simulink library "tqd"  (R2021b)
settings: Solver=VariableStepAuto  StartTime=0.0  StopTime=10.0  RelTol=1e-3
undefined symbols (not defined in the file or in its folder): ATQD_APSDecReq_X_kph, ATQD_APSDecReq_Y_mps2, ATQD_APSDecReqCMD_X_kph, ATQD_APSDecReqTs_X_pct, ATQD_APSDecTimeGain_X_Deg, ATQD_APSDecTimeGain_Y_s, ATQD_APSReqLowSpd_X_Deg, ATQD_AutoHoldReleaseBPS_X_Deg, ATQD_AWDLoadTrqnsGain_X_kg, ATQD_AWDLoadTrqnsGain_Y_pct, ATQD_BOSEnBPSPosn_X_kph, ATQD_BOSMap_X_rpm, ATQD_BOSMap_Y_pct, ATQD_CreepBaseTqD_X_kph, ATQD_CreepBaseTqD_Y_Deg, ATQD_CreepBaseTqR_X_kph, ATQD_CreepBaseTqR_Y_Deg, ATQD_CreepBPSDisPosn_X_Deg, ATQD_CreepBPSDisPosnR_X_Deg, ATQD_CreepBPSEnPosn_X_Deg, ATQD_CreepBPSEnPosnR_X_Deg, ATQD_CreepDeltaTq_X_kph, ATQD_CreepIterm_X_kph, ATQD_CreepIterm_Y_kph, ATQD_CreepItermMaxLimit_X_pct, ATQD_CreepPreloadTime_X_kph, ATQD_CreepPreloadTq_X_kph, ATQD_CreepPreloadTq_Y_s, ATQD_CreepProtTq_X_Deg, ATQD_CreepPterm_X_kph, ATQD_ECOTqMapD_X_rpm, ATQD_ECOTqMapD_Y_pct, ATQD_EOPDTqMapDCon_X_rpm, ATQD_EOPDTqMapDCon_Y_Deg, ATQD_EstInitVehWeight_X_c, ATQD_LHMRollGenMapD_X_rpm, ATQD_LHMRollGenMapD_Y_rpm, ATQD_LHMTqMapD_X_rpm, ATQD_LHMTqMapD_Y_pct, ATQD_NL1TqMapD_X_rpm, ATQD_NL1TqMapD_Y_pct, ATQD_NOPDTqMapDCon_X_rpm, ATQD_NOPDTqMapDCon_Y_Deg, ATQD_NRMRrEDUSpRat_X_rpm, ATQD_NRMRrEDUSpRat_Y_Nm, ATQD_OPDHoldDownRelDelay_X_Deg, ATQD_OPDHoldEnSpd_X_Deg, ATQD_OPDHoldRelDetTime_X_Deg, ATQD_OPDHoldReleaseTq_X_Deg, ATQD_OrigPedTqLowLim_X_Deg, ATQD_OrigPedTqLowLim_Y_pct, ATQD_PedalMapClimbUpLim_X_rpm, ATQD_PedalMapClimbUpLim_Y_Deg, ATQD_PreLoadTq_X_s, ATQD_RollGenMapEL1_X_rpm, ATQD_RollGenMapEL1_Y_rpm, ATQD_SL1TqMapD_X_rpm, ATQD_SL1TqMapD_Y_pct, ATQD_SlideRegenTqGain_X_Gps, ATQD_SlideRegenTqGain_Y_pct ... (+378)
libraries: hcu_lib x59, simulink x49
(part 2 of 12)

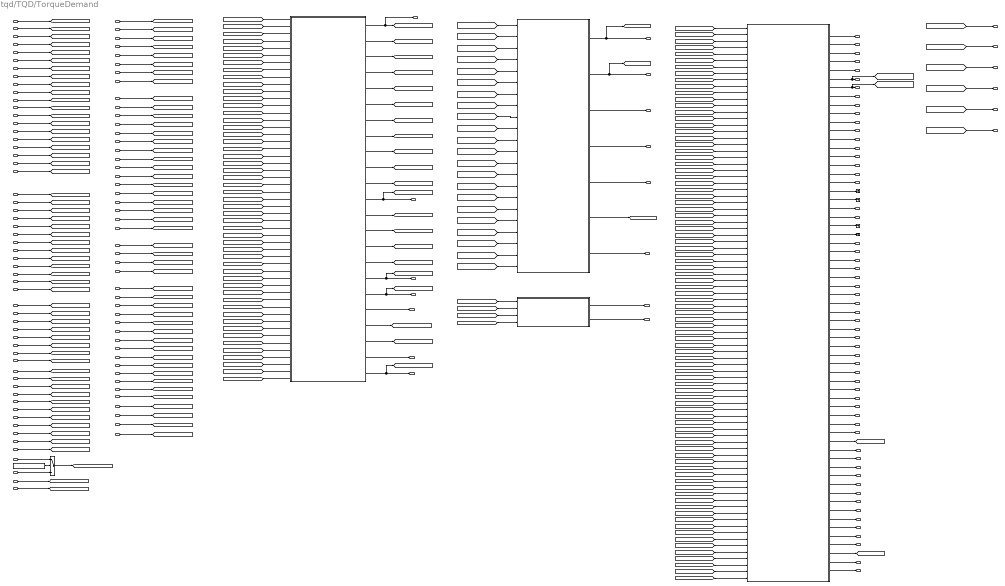
== system tqd/TQD/TorqueDemand ==
  note: Input Signals
  task_time_s : Inport
  VDHP_ActAPSPosn_pct : Inport  Port=2
  VDHP_LowIdleAccPedal_flg : Inport  Port=3
  VPMM_PowerSta_enum : Inport  Port=4
  VPMM_DrivetrainSelect_enum : Inport  Port=5
  VPMM_SysPowerMode_enum : Inport  Port=6
  VINP_VehSpeed_kph : Inport  Port=7
  VINP_BrkSwSta_flg : Inport  Port=8
  VINP_BrkSwV_flg : Inport  Port=9
  VINP_BrkPedalPos_pct : Inport  Port=10
  VINP_BrkPedalPosSta_flg : Inport  Port=11
  VINP_FrPTCSActive_flg : Inport  Port=12
  VINP_RrPTCSActive_flg : Inport  Port=13
  VINP_FrntAxlTrqReqDrv_Nm : Inport  Port=14
  VINP_RearAxlTrqReqDrv_Nm : Inport  Port=15
  VINP_FrRBCActive_flg : Inport  Port=16
  VINP_RrRBCActive_flg : Inport  Port=17
  VINP_FrntAxlTrqReqBrk_Nm : Inport  Port=18
  VINP_RearAxlTrqReqBrk_Nm : Inport  Port=19
  VINP_ADASForceIdle_flg : Inport  Port=20
  VINP_CrashOutputSts_enum : Inport  Port=21
  VINP_LongAccel_Gps : Inport  Port=22
  VINP_EPBCarWashMode_flg : Inport  Port=23
  VINP_EPBErrSta_enum : Inport  Port=24
  VINP_EPBSta_enum : Inport  Port=25
  VINP_DOASta_flg : Inport  Port=26
  VINP_HSAActive_flg : Inport  Port=27
  VINP_DriverSeatBeltCmd_flg : Inport  Port=28
  VINP_AVHActive_flg : Inport  Port=29
  VINP_ACCRequiredAccel_mps2 : Inport  Port=30
  VINP_ACCVehHoldReq_flg : Inport  Port=31
  VINP_PsngrSeatBeltCmd_flg : Inport  Port=32
  VINP_RDriverSeatBeltCmd_flg : Inport  Port=33
  VINP_RCenterSeatBeltCmd_flg : Inport  Port=34
  VINP_RPsngrSeatBeltCmd_flg : Inport  Port=35
  VINP_SASAngle_Deg : Inport  Port=36
  VINP_YawRate_degps : Inport  Port=37
  VINP_ADASACCSta_enum : Inport  Port=38
  VINP_ABSActive_flg : Inport  Port=39
  VINP_ESCActive_flg : Inport  Port=40
  VINP_IVIPWModeReq_enum : Inport  Port=41
  VINP_IVICreepSWReq_flg : Inport  Port=42
  VINP_RollModeSWCmd_enum : Inport  Port=43
  VINP_IVIPwrLockSW_enum : Inport  Port=44
  VINP_ShifterHandleCmd_enum : Inport  Port=45
  VINP_FrEDURotateDirction_enum : Inport  Port=46
  VINP_RrEDURotateDirction_enum : Inport  Port=47
  VINP_FrTMSpd_RPM : Inport  Port=48
  VINP_RrTMSpd_RPM : Inport  Port=49
  VINP_HVBPwrAvailDchrg_kw : Inport  Port=50
  VINP_HVBPwrAvailChrg_kw : Inport  Port=51
  VINP_FrRegenAvailTq_Nm : Inport  Port=52
  VINP_RrRegenAvailTq_Nm : Inport  Port=53
  VINP_FrEDURealTMTq_Nm : Inport  Port=54
  VINP_RrEDURealTMTq_Nm : Inport  Port=55
  VINP_HVBattErr_flg : Inport  Port=56
  VINP_DCDCFaultSta_enum : Inport  Port=57
  VINP_FrMotorAvailTq_Nm : Inport  Port=58
  VINP_RrMotorAvailTq_Nm : Inport  Port=59
  VINP_MCUWarnF_enum : Inport  Port=60
  VINP_MCUWarnR_enum : Inport  Port=61
  VINP_ChrgPlugSta_enum : Inport  Port=62
  VINP_HVBattSOC_pct : Inport  Port=63
  VINP_RegenMode_enum : Inport  Port=64
  VINP_DrSCPSysErrLmp_enum : Inport  Port=65
  VINP_SCPSystemMode_enum : Inport  Port=66
  VVMC_ADASActive_flg : Inport  Port=67
  VVMC_ADASWhlTqReq_Nm : Inport  Port=68
  VVMC_CruzActive_flg : Inport  Port=69
  VVMC_CruzWhlTqReq_Nm : Inport  Port=70
  VVMC_MSAActive_flg : Inport  Port=71
  VVMC_MSAWhlTqReq_Nm : Inport  Port=72
  VVMC_APSActive_flg : Inport  Port=73
  VVMC_APSSpeedCMD_kph : Inport  Port=74
  VVMC_APSShiftPosnReq_enum : Inport  Port=75
  VVMC_ACCPedalOvrd_flg : Inport  Port=76
  VVMC_LongAcc_Gps : Inport  Port=77
  VVMC_ActMaxSlideRate_pct : Inport  Port=78
  VVMC_EstSlope_Deg : Inport  Port=79
  VVMC_APSReq_enum : Inport  Port=80
  VVMC_RWDRDCActive_enum : Inport  Port=81
  VVMC_ActLRSlideRate_pct : Inport  Port=82
  VVMC_ActRRSlideRate_pct : Inport  Port=83
  VVMC_ActStESCYaw_degps : Inport  Port=84
  VVMC_CAASActive_flg : Inport  Port=85
  VVMC_CalibratedGyroY_Dps : Inport  Port=86
  VINP_BrakeSWGPIO_flg : Inport  Port=87
  VINP_CrashSignalGPIO_flg : Inport  Port=88
  VINP_DrDoorSW_flg : Inport  Port=89
  VINP_SeatSW_flg : Inport  Port=90
  VINP_HoodSW_flg : Inport  Port=91
  VINP_TailgateSW_flg : Inport  Port=92
  VINP_PsDoorSW_flg : Inport  Port=93
  VINP_RRDoorSW_flg : Inport  Port=94
  VINP_RLDoorSW_flg : Inport  Port=95
  VTQR_ActualFEDUWhlTqReq_Nm : Inport  Port=96
  VTQR_ActualREDUWhlTqReq_Nm : Inport  Port=97
  VTQR_NoABSFEDUWhlTqReq_Nm : Inport  Port=98
  VTQR_NoABSREDUWhlTqReq_Nm : Inport  Port=99
  VINP_PBWMotorPos_enum : Inport  Port=100
  VDDM_LimpHomeAct_flg : Inport  Port=101
  VINP_CreepSW_flg : Inport  Port=102
  Constant21 : Constant  Value=KTQD_YawRateSW_flg
  CrashDetect : Subsystem
  ShiftModule : Subsystem
      settings: AttributesFormatString=Priority%<Priority>
  Signal_convert : Subsystem
  Switch : Switch  Criteria=u2 > Threshold
  Terminator{,1..3} (4 alike) : Terminator
  TorqueModule : Subsystem
      settings: AttributesFormatString=Priority%<Priority>
  VTQD_GearActualPosn_enum : Outport
  VTQD_ParkRequest_flg : Outport  Port=2
  VTQD_PBWLockTO_flg : Outport  Port=3
  VTQD_PBWUnlockTO_flg : Outport  Port=4
  VTQD_DriverWhlTqDem_Nm : Outport  Port=5
  VTQD_AfterAvailableTqDemFr_Nm : Outport  Port=6
  VTQD_AfterAvailableTqDemRr_Nm : Outport  Port=7
  VTQD_TqSourceFr_enum : Outport  Port=8
  VTQD_TqSourceRr_enum : Outport  Port=9
  VTQD_FrEDUAvailBrkRgnTq_Nm : Outport  Port=10
  VTQD_RrEDUAvailBrkRgnTq_Nm : Outport  Port=11
  VTQD_TqTargetShaftSpd_rpm : Outport  Port=12
  VTQD_LimpHomeAct_flg : Outport  Port=13
  VTQD_RollRegenEnable_flg : Outport  Port=14
  VTQD_EVDriveMode_enum : Outport  Port=15
  VTQD_EVDriveModeValid_flg : Outport  Port=16
  VTQD_ShiftGearPosn_enum : Outport  Port=17
  VTQD_PButtonSta_enum : Outport  Port=18
  VTQD_FrActvDmpDisabReq_flg : Outport  Port=19
  VTQD_RrActvDmpDisabReq_flg : Outport  Port=20
  VTQD_FrRgnDecrSta_flg : Outport  Port=21
  VTQD_RrRgnDecrSta_flg : Outport  Port=22
  VTQD_DriverWhlTqDemFr_Nm : Outport  Port=23
  VTQD_DriverWhlTqDemRr_Nm : Outport  Port=24
  VTQD_FrEDUActTq_Nm : Outport  Port=25
  VTQD_RrEDUActTq_Nm : Outport  Port=26
  VTQD_FrEDURolRgnTq_Nm : Outport  Port=27
  VTQD_RrEDURolRgnTq_Nm : Outport  Port=28
  VTQD_FrEDUSpd_rpm : Outport  Port=29
  VTQD_RrEDUSpd_rpm : Outport  Port=30
  VTQD_FrEDUSpdValid_flg : Outport  Port=31
  VTQD_FrEDUAvailBrkRgnTqV_flg : Outport  Port=32
  VTQD_RrEDUSpdValid_flg : Outport  Port=33
  VTQD_RrEDUAvailBrkRgnTqV_flg : Outport  Port=34
  VTQD_RgnAbnorSta_flg : Outport  Port=35
  VTQD_PTCSPermSta_flg : Outport  Port=36
  VTQD_FrRgnPermSta_flg : Outport  Port=37
  VTQD_RrRgnPermSta_flg : Outport  Port=38
  VTQD_ExternalTqAllow_flg : Outport  Port=39
  VTQD_FrIdcMin_A : Outport  Port=40
  VTQD_FrIdcMax_A : Outport  Port=41
  VTQD_FrUdcMin_V : Outport  Port=42
  VTQD_FrUdcMax_V : Outport  Port=43
  VTQD_RrIdcMin_A : Outport  Port=44
  VTQD_RrIdcMax_A : Outport  Port=45
  VTQD_RrUdcMin_V : Outport  Port=46
  VTQD_RrUdcMax_V : Outport  Port=47
  VTQD_CoordWhlTqDemFr_Nm : Outport  Port=48
  VTQD_CoordWhlTqDemRr_Nm : Outport  Port=49
  VTQD_CreepEnable_flg : Outport  Port=50
  VTQD_CrashDetd_flg : Outport  Port=51
  VTQD_DiagHCrash_flg : Outport  Port=52
  VTQD_ReBrakeLPReq_flg : Outport  Port=53
  VTQD_LoSpdBrkCtrl_flg : Outport  Port=54
  VTQD_LowIdleAccPedal_flg : Outport  Port=55
  VTQD_APSStaSys_enum : Outport  Port=56
  VTQD_APSReq_enum : Outport  Port=57
  VTQD_APSDecReqA_flg : Outport  Port=58
  VTQD_APSDecReq_mps2 : Outport  Port=59
  VTQD_ExtShftAllow_flg : Outport  Port=60
  VTQD_EstVehWeightResult_kg : Outport  Port=61
  VTQD_BOSEnable_flg : Outport  Port=62
  VTQD_CreepON_flg : Outport  Port=63
  VTQD_PreLoadHold_flg : Outport  Port=64
  VTQD_PreLoadPreEn_flg : Outport  Port=65
  VTQD_CreepPrLoadEnable_flg : Outport  Port=66
  VTQD_RDCActive_enum : Outport  Port=67
  VTQD_EquivAccPedalSWSta_flg : Outport  Port=68
  VTQD_DriveProtEn_flg : Outport  Port=69
  VTQD_ActParkRequest_flg : Outport  Port=70
  VTQD_RegenTqLimitEn_flg : Outport  Port=71
  VTQD_PedAccTqEn_flg : Outport  Port=72
  VTQD_IVIPwrLockSta_enum : Outport  Port=73
  VTQD_ExtDoorAllow_flg : Outport  Port=74
  VTQD_OPDHoldLamp_flg : Outport  Port=75
  VTQD_RegenMode_enum : Outport  Port=76
  VTQD_VehActSpd_kph : Outport  Port=77
  VTQD_CreepBaseTqD_Nm : Outport  Port=78
  wires:
  VINP_FrTMSpd_RPM/1 -> [VINP_FrTMSpd_rpm]
  VDHP_ActAPSPosn_pct/1 -> [VDHP_ActAPSPosn_pct]
  VPMM_PowerSta_enum/1 -> [VPMM_PowerSta_enum]
  task_time_s/1 -> [task_time_s]
  VINP_VehSpeed_kph/1 -> [VINP_VehSpeed_kph]
  VINP_BrkSwSta_flg/1 -> [VINP_BrkSwSta_flg]
  VINP_ShifterHandleCmd_enum/1 -> [VINP_ShifterHandleCmd_enum]
  VDHP_LowIdleAccPedal_flg/1 -> [VDHP_LowIdleAccPedal_flg]
  VINP_PBWMotorPos_enum/1 -> [VINP_PBWMotorPos_enum]
  Signal_convert/8(VTQD_TqTargetShaftSpd_rpm) -> [VTQD_TqTargetShaftSpd_rpm]
  Signal_convert/2(VTQD_RollRegenDisable_flg) -> [VTQD_RollRegenDisableReq_flg]
  Signal_convert/5(VTQD_ActBPSPosn_pct) -> [VTQD_ActBPSPosn_pct]
  Signal_convert/11(VTQD_EVDriveMode_enum) -> [VTQD_EVDriveMode_enum]
  Signal_convert/10(VTQD_LimpHomeAct_flg) -> [VTQD_LimpHomeAct_flg]
  Signal_convert/12(VTQD_CreepON_flg) -> [VTQD_CreepON_flg], VTQD_CreepON_flg/1
  [VTQD_TMRotateDirction_enum] -> ShiftModule/7(VTQD_TMRotateDirction_enum)
  ShiftModule/4(VTQD_PBWUnlockTO_flg) -> VTQD_PBWUnlockTO_flg/1
  [VINP_VehSpeed_kph] -> ShiftModule/3(VINP_VehSpeed_kph)
  [VPMM_PowerSta_enum] -> ShiftModule/5(VPMM_PowerSta_enum)
  [task_time_s] -> ShiftModule/1(task_time_s)
  [VTQD_BrkSwSta_flg] -> ShiftModule/4(VTQD_BrkSwSta_flg)
  ShiftModule/2(VTQD_ParkRequest_flg) -> [VTQD_ParkRequest_flg], VTQD_ParkRequest_flg/1
  [VINP_ShifterHandleCmd_enum] -> ShiftModule/2(VINP_ShifterHandleCmd_enum)
  ShiftModule/3(VTQD_PBWLockTO_flg) -> VTQD_PBWLockTO_flg/1
  [VINP_PBWMotorPos_enum] -> ShiftModule/6(VINP_PBWMotorPos_enum)
  ShiftModule/1(VTQD_GearActualPosn_enum) -> [VTQD_GearActualPosn_enum], VTQD_GearActualPosn_enum/1
  [VTQD_RollRegenDisableReq_flg] -> TorqueModule/3(VTQD_RollRegenDisableReq_flg)
  [VTQD_GearActualPosn_enum] -> TorqueModule/4(VTQD_GearActualPosn_enum)
  [VTQD_CreepON_flg] -> TorqueModule/5(VTQD_CreepON_flg)
  [VTQD_BrkSwSta_flg] -> TorqueModule/6(VTQD_BrkSwSta_flg)
  [VINP_FrntAxlTrqReqBrk_Nm] -> TorqueModule/22(VINP_FrntAxlTrqReqBrk_Nm)
  [VINP_RearAxlTrqReqBrk_Nm] -> TorqueModule/23(VINP_RearAxlTrqReqBrk_Nm)
  [VINP_RearAxlTrqReqDrv_Nm] -> TorqueModule/19(VINP_RearAxlTrqReqDrv_Nm)
  [VINP_FrntAxlTrqReqDrv_Nm] -> TorqueModule/18(VINP_FrntAxlTrqReqDrv_Nm)
  [VTQD_LimpHomeAct_flg] -> TorqueModule/7(VTQD_LimpHomeAct_flg)
  [VINP_VehSpeed_kph] -> TorqueModule/10(VINP_VehSpeed_kph)
  [VTQD_TqTargetShaftSpd_rpm] -> TorqueModule/11(VTQD_TqTargetShaftSpd_rpm)
  [VTQD_ActBPSPosn_pct] -> TorqueModule/15(VTQD_ActBPSPosn_pct)
  [VVMC_APSActive_flg] -> TorqueModule/30(VVMC_APSActive_flg)
  [VVMC_ADASActive_flg] -> TorqueModule/24(VVMC_ADASActive_flg)
  [VVMC_ADASWhlTqReq_Nm] -> TorqueModule/25(VVMC_ADASWhlTqReq_Nm)
  [VVMC_CruzActive_flg] -> TorqueModule/26(VVMC_CruzActive_flg)
  [VVMC_CruzWhlTqReq_Nm] -> TorqueModule/27(VVMC_CruzWhlTqReq_Nm)
  [VVMC_MSAActive_flg] -> TorqueModule/28(VVMC_MSAActive_flg)
  [VVMC_MSAWhlTqReq_Nm] -> TorqueModule/29(VVMC_MSAWhlTqReq_Nm)
  VINP_HVBPwrAvailDchrg_kw/1 -> [VINP_HVBPwrAvailDchrg_kw]
  VINP_HVBPwrAvailChrg_kw/1 -> [VINP_HVBPwrAvailChrg_kw]
  [VINP_HVBPwrAvailDchrg_kw] -> TorqueModule/31(VINP_HVBPwrAvailDchrg_kw)
  [VINP_HVBPwrAvailChrg_kw] -> TorqueModule/34(VINP_HVBPwrAvailChrg_kw)
  [VINP_CreepSW_flg] -> Signal_convert/15(VINP_CreepSW_flg)
  VINP_CreepSW_flg/1 -> [VINP_CreepSW_flg]
  VDDM_LimpHomeAct_flg/1 -> [VDDM_LimpHomeAct_flg]
  [VDDM_LimpHomeAct_flg] -> Signal_convert/14(VDDM_LimpHomeAct_flg)
  VINP_BrkSwV_flg/1 -> [VINP_BrkSwV_flg]
  VINP_FrPTCSActive_flg/1 -> [VINP_FrPTCSActive_flg]
  VINP_FrntAxlTrqReqDrv_Nm/1 -> [VINP_FrntAxlTrqReqDrv_Nm]
  VINP_RearAxlTrqReqDrv_Nm/1 -> [VINP_RearAxlTrqReqDrv_Nm]
  VINP_FrRBCActive_flg/1 -> [VINP_FrRBCActive_flg]
  VINP_FrntAxlTrqReqBrk_Nm/1 -> [VINP_FrntAxlTrqReqBrk_Nm]
  VINP_RearAxlTrqReqBrk_Nm/1 -> [VINP_RearAxlTrqReqBrk_Nm]
  VINP_BrkPedalPos_pct/1 -> [VINP_BrkPedalPos_pct]
  VINP_BrkPedalPosSta_flg/1 -> [VINP_BrkPedalPosSta_flg]
  [VINP_BrkSwSta_flg] -> Signal_convert/4(VINP_BrkSwSta_flg)
  [VINP_BrkSwV_flg] -> Signal_convert/6(VINP_BrkSwV_flg)
  [VINP_BrkPedalPos_pct] -> Signal_convert/7(VINP_BrkPedalPos_pct)
  [VINP_BrkPedalPosSta_flg] -> Signal_convert/8(VINP_BrkPedalPosSta_flg)
  [VTQD_TqTargetShaftSpd_rpm] -> VTQD_TqTargetShaftSpd_rpm/1
  [VTQD_LowIdleAccPedal_flg] -> TorqueModule/1(VTQD_LowIdleAccPedal_flg)
  [VPMM_DrivetrainSelect_enum] -> TorqueModule/2(VPMM_DrivetrainSelect_enum)
  VINP_RrTMSpd_RPM/1 -> [VINP_RrTMSpd_rpm]
  [VPMM_DrivetrainSelect_enum] -> Signal_convert/11(VPMM_DrivetrainSelect_enum)
  VPMM_DrivetrainSelect_enum/1 -> [VPMM_DrivetrainSelect_enum]
  [VDHP_ActAPSPosn_pct] -> Signal_convert/3(VDHP_ActAPSPosn_pct)
  Signal_convert/3(VTQD_ActAPSPosn_pct) -> [VTQD_ActAPSPosn_pct]
  [VTQD_ActAPSPosn_pct] -> TorqueModule/14(VTQD_ActAPSPosn_pct)
  [VTQD_GearActualPosn_enum] -> Signal_convert/1(VTQD_GearActualPosn_enum)
  [VINP_FrTMSpd_rpm] -> Signal_convert/9(VINP_FrTMSpd_rpm)
  [VINP_RrTMSpd_rpm] -> Signal_convert/10(VINP_RrTMSpd_rpm)
  VINP_FrEDURotateDirction_enum/1 -> [VINP_FrEDURotateDirction_enum]
  VINP_RrEDURotateDirction_enum/1 -> [VINP_RrEDURotateDirction_enum]
  [VINP_RrEDURotateDirction_enum] -> Signal_convert/13(VINP_RrEDURotateDirction_enum)
  [VINP_FrEDURotateDirction_enum] -> Signal_convert/12(VINP_FrEDURotateDirction_enum)
  Signal_convert/6(VTQD_FrShaftSpd_rpm) -> [VTQD_FrShaftSpd_rpm]
  Signal_convert/7(VTQD_RrShaftSpd_rpm) -> [VTQD_RrShaftSpd_rpm]
  Signal_convert/9(VTQD_TMRotateDirction_enum) -> [VTQD_TMRotateDirction_enum]
  Signal_convert/4(VTQD_BrkSwSta_flg) -> [VTQD_BrkSwSta_flg]
  [VTQD_FrShaftSpd_rpm] -> TorqueModule/12(VTQD_FrShaftSpd_rpm)
  [VTQD_RrShaftSpd_rpm] -> TorqueModule/13(VTQD_RrShaftSpd_rpm)
  Signal_convert/1(VTQD_LowIdleAccPedal_flg) -> VTQD_LowIdleAccPedal_flg/1, [VTQD_LowIdleAccPedal_flg]
  [VDHP_LowIdleAccPedal_flg] -> Signal_convert/2(VDHP_LowIdleAccPedal_flg)
  [VTQD_LimpHomeAct_flg] -> VTQD_LimpHomeAct_flg/1
  [VTQD_EVDriveMode_enum] -> VTQD_EVDriveMode_enum/1
  VINP_BrakeSWGPIO_flg/1 -> [VINP_BrakeSWGPIO_flg]
  [VINP_BrakeSWGPIO_flg] -> Signal_convert/5(VINP_BrakeSWGPIO_flg)
  Signal_convert/13(VTQD_ShiftGearPosn_enum) -> [VTQD_ShiftGearPosn_enum]
  [VTQD_ShiftGearPosn_enum] -> VTQD_ShiftGearPosn_enum/1
  ShiftModule/5(VTQD_PButtonSta_enum) -> VTQD_PButtonSta_enum/1
  [VINP_VehSpeed_kph] -> Signal_convert/16(VINP_VehSpeed_kph)
  Signal_convert/14(VTQD_FrActvDmpDisabReq_flg) -> [VTQD_FrActvDmpDisabReq_flg]
  Signal_convert/15(VTQD_RrActvDmpDisabReq_flg) -> [VTQD_RrActvDmpDisabReq_flg]
  [VTQD_FrActvDmpDisabReq_flg] -> VTQD_FrActvDmpDisabReq_flg/1
  [VTQD_RrActvDmpDisabReq_flg] -> VTQD_RrActvDmpDisabReq_flg/1
  VINP_RrPTCSActive_flg/1 -> [VINP_RrPTCSActive_flg]
  [VINP_FrPTCSActive_flg] -> TorqueModule/16(VINP_FrPTCSActive_flg)
  [VINP_RrPTCSActive_flg] -> TorqueModule/17(VINP_RrPTCSActive_flg)
  VINP_RrRBCActive_flg/1 -> [VINP_RrRBCActive_flg]
  [VINP_FrRBCActive_flg] -> TorqueModule/20(VINP_FrRBCActive_flg)
  [VINP_RrRBCActive_flg] -> TorqueModule/21(VINP_RrRBCActive_flg)
  VINP_RrRegenAvailTq_Nm/1 -> [VINP_RrRegenAvailTq_Nm]
  VINP_FrEDURealTMTq_Nm/1 -> [VINP_FrEDURealTMTq_Nm]
  VINP_FrRegenAvailTq_Nm/1 -> [VINP_FrRegenAvailTq_Nm]
  VINP_RrEDURealTMTq_Nm/1 -> [VINP_RrEDURealTMTq_Nm]
  [VINP_FrRegenAvailTq_Nm] -> TorqueModule/35(VINP_FrRegenAvailTq_Nm)
  [VINP_RrRegenAvailTq_Nm] -> TorqueModule/36(VINP_RrRegenAvailTq_Nm)
  [VINP_FrTMSpd_rpm] -> TorqueModule/37(VINP_FrTMSpd_RPM)
  [VINP_RrTMSpd_rpm] -> TorqueModule/38(VINP_RrTMSpd_RPM)
  [VINP_FrEDURealTMTq_Nm] -> TorqueModule/39(VINP_FrEDURealTMTq_Nm)
  [VINP_RrEDURealTMTq_Nm] -> TorqueModule/40(VINP_RrEDURealTMTq_Nm)
  [VTQD_ParkRequest_flg] -> TorqueModule/41(VTQD_ParkRequest_flg)
  Signal_convert/16(VTQD_MCUReady4Ext_flg) -> [VTQD_MCUReady4Ext_flg]
  [VPMM_PowerSta_enum] -> TorqueModule/42(VPMM_PwrSta_enum)
  [VTQD_MCUReady4Ext_flg] -> TorqueModule/43(VTQD_MCUReady4Ext_flg)
  VINP_DCDCFaultSta_enum/1 -> [VINP_DCDCFaultSta_enum]
  VINP_ADASForceIdle_flg/1 -> [VINP_ADASForceIdle_flg]
  VINP_HVBattErr_flg/1 -> [VINP_HVBattErr_flg]
  [VINP_HVBattErr_flg] -> TorqueModule/44(VINP_HVBattErr_flg)
  [VINP_DCDCFaultSta_enum] -> TorqueModule/45(VINP_DCDCFaultSta_enum)
  [VINP_ADASForceIdle_flg] -> TorqueModule/46(VINP_ADASForceIdle_flg)
  VVMC_ADASActive_flg/1 -> [VVMC_ADASActive_flg]
  VVMC_ADASWhlTqReq_Nm/1 -> [VVMC_ADASWhlTqReq_Nm]
  VVMC_APSActive_flg/1 -> [VVMC_APSActive_flg]
  [VTQD_TMRotateDirction_enum] -> TorqueModule/47(VTQD_TMRotateDirction_enum)
  VINP_IVIPWModeReq_enum/1 -> [VINP_IVIPWModeReq_enum]
  VINP_RegenMode_enum/1 -> [VINP_RegenMode_enum]
  [VTQD_EVDriveMode_enum] -> TorqueModule/8(VTQD_EVDriveMode_enum)
  [VTQD_RegenMode_enum] -> TorqueModule/9(VTQD_RegenMode_enum)
  TorqueModule/1(VTQD_DriverWhlTqDem_Nm) -> VTQD_DriverWhlTqDem_Nm/1
  TorqueModule/2(VTQD_TqSourceFr_enum) -> VTQD_TqSourceFr_enum/1
  TorqueModule/3(VTQD_TqSourceRr_enum) -> VTQD_TqSourceRr_enum/1  "VTQD_TqSourceRr_enum"
  TorqueModule/4(VTQD_RollRegenEnable_flg) -> VTQD_RollRegenEnable_flg/1
  TorqueModule/5(VTQD_EVDriveModeValid_flg) -> VTQD_EVDriveModeValid_flg/1
  TorqueModule/6(VTQD_AfterAvailableTqDemFr_Nm) -> [VTQD_AfterAvailableTqDemFr_Nm], VTQD_AfterAvailableTqDemFr_Nm/1
  TorqueModule/7(VTQD_AfterAvailableTqDemRr_Nm) -> [VTQD_AfterAvailableTqDemRr_Nm], VTQD_AfterAvailableTqDemRr_Nm/1
  TorqueModule/8(VTQD_FrEDUAvailBrkRgnTq_Nm) -> VTQD_FrEDUAvailBrkRgnTq_Nm/1
  TorqueModule/9(VTQD_RrEDUAvailBrkRgnTq_Nm) -> VTQD_RrEDUAvailBrkRgnTq_Nm/1
  TorqueModule/10(VTQD_FrRgnDecrSta_flg) -> VTQD_FrRgnDecrSta_flg/1
  TorqueModule/11(VTQD_RrRgnDecrSta_flg) -> VTQD_RrRgnDecrSta_flg/1
  TorqueModule/12(VTQD_FrEDUActTq_Nm) -> VTQD_FrEDUActTq_Nm/1
  TorqueModule/13(VTQD_RrEDUActTq_Nm) -> VTQD_RrEDUActTq_Nm/1
  TorqueModule/14(VTQD_FrEDURolRgnTq_Nm) -> VTQD_FrEDURolRgnTq_Nm/1
  TorqueModule/15(VTQD_RrEDURolRgnTq_Nm) -> VTQD_RrEDURolRgnTq_Nm/1
  TorqueModule/16(VTQD_FrEDUSpd_rpm) -> VTQD_FrEDUSpd_rpm/1
  TorqueModule/17(VTQD_RrEDUSpd_rpm) -> VTQD_RrEDUSpd_rpm/1
  TorqueModule/18(VTQD_FrEDUSpdValid_flg) -> VTQD_FrEDUSpdValid_flg/1
  TorqueModule/21(VTQD_FrEDUAvailBrkRgnTqV_flg) -> VTQD_FrEDUAvailBrkRgnTqV_flg/1
  TorqueModule/22(VTQD_RrEDUSpdValid_flg) -> VTQD_RrEDUSpdValid_flg/1
  TorqueModule/23(VTQD_RrEDUActTqValid_flg) -> Terminator2/1
  TorqueModule/24(VTQD_RrEDURolRgnTqValid_flg) -> Terminator3/1
  TorqueModule/25(VTQD_RrEDUAvailBrkRgnTqV_flg) -> VTQD_RrEDUAvailBrkRgnTqV_flg/1
  TorqueModule/26(VTQD_RgnAbnorSta_flg) -> VTQD_RgnAbnorSta_flg/1
  TorqueModule/27(VTQD_PTCSPermSta_flg) -> VTQD_PTCSPermSta_flg/1
  TorqueModule/28(VTQD_FrRgnPermSta_flg) -> VTQD_FrRgnPermSta_flg/1
  TorqueModule/29(VTQD_RrRgnPermSta_flg) -> VTQD_RrRgnPermSta_flg/1
  TorqueModule/30(VTQD_DriverWhlTqDemFr_Nm) -> VTQD_DriverWhlTqDemFr_Nm/1
  TorqueModule/31(VTQD_DriverWhlTqDemRr_Nm) -> VTQD_DriverWhlTqDemRr_Nm/1
  TorqueModule/32(VTQD_ExternalTqAllow_flg) -> VTQD_ExternalTqAllow_flg/1
  TorqueModule/33(VTQD_FrIdcMin_A) -> VTQD_FrIdcMin_A/1
  TorqueModule/34(VTQD_FrIdcMax_A) -> VTQD_FrIdcMax_A/1
  TorqueModule/35(VTQD_FrUdcMin_V) -> VTQD_FrUdcMin_V/1
  TorqueModule/36(VTQD_FrUdcMax_V) -> VTQD_FrUdcMax_V/1
  TorqueModule/37(VTQD_RrIdcMin_A) -> VTQD_RrIdcMin_A/1
  TorqueModule/38(VTQD_RrIdcMax_A) -> VTQD_RrIdcMax_A/1
  TorqueModule/39(VTQD_RrUdcMin_V) -> VTQD_RrUdcMin_V/1
  TorqueModule/40(VTQD_RrUdcMax_V) -> VTQD_RrUdcMax_V/1
  TorqueModule/41(VTQD_CoordWhlTqDemFr_Nm) -> VTQD_CoordWhlTqDemFr_Nm/1
  TorqueModule/42(VTQD_CoordWhlTqDemRr_Nm) -> VTQD_CoordWhlTqDemRr_Nm/1
  TorqueModule/43(VTQD_CreepEnable_flg) -> VTQD_CreepEnable_flg/1
  [VINP_IVIPWModeReq_enum] -> Signal_convert/17(VINP_IVIPWModeReq_enum)
  VVMC_CruzActive_flg/1 -> [VVMC_CruzActive_flg]
  VVMC_CruzWhlTqReq_Nm/1 -> [VVMC_CruzWhlTqReq_Nm]
  VVMC_MSAActive_flg/1 -> [VVMC_MSAActive_flg]
  VVMC_MSAWhlTqReq_Nm/1 -> [VVMC_MSAWhlTqReq_Nm]
  VINP_CrashSignalGPIO_flg/1 -> [VINP_CrashSignalGPIO_flg]
  VINP_CrashOutputSts_enum/1 -> [VINP_CrashOutputSts_enum]
  CrashDetect/1(VTQD_CrashDetd_flg) -> VTQD_CrashDetd_flg/1  "VTQD_CrashDetd_flg"
  CrashDetect/2(VTQD_DiagHCrash_flg) -> VTQD_DiagHCrash_flg/1  "VTQD_DiagHCrash_flg"
  VINP_LongAccel_Gps/1 -> [VINP_LongAccel_Gps]
  [VINP_LongAccel_Gps] -> TorqueModule/48(VINP_LongAccel_Gps)
  TorqueModule/44(VTQD_ReBrakeLPReq_flg) -> VTQD_ReBrakeLPReq_flg/1
  VTQR_ActualFEDUWhlTqReq_Nm/1 -> [VTQR_ActualFEDUWhlTqReq_Nm]
  VTQR_ActualREDUWhlTqReq_Nm/1 -> [VTQR_ActualREDUWhlTqReq_Nm]
  [VTQR_ActualFEDUWhlTqReq_Nm] -> TorqueModule/49(VTQR_ActualFEDUWhlTqReq_Nm)
  [VTQR_ActualREDUWhlTqReq_Nm] -> TorqueModule/50(VTQR_ActualREDUWhlTqReq_Nm)
  [VTQD_RDCActive_enum] -> TorqueModule/51(VTQD_RDCActive_enum)
  VINP_EPBCarWashMode_flg/1 -> [VINP_EPBCarWashMode_flg]
  VINP_EPBErrSta_enum/1 -> [VINP_EPBErrSta_enum]
  VINP_EPBSta_enum/1 -> [VINP_EPBSta_enum]
  VINP_DOASta_flg/1 -> [VINP_DOASta_flg]
  VINP_FrMotorAvailTq_Nm/1 -> [VINP_FrMotorAvailTq_Nm]
  VINP_RrMotorAvailTq_Nm/1 -> [VINP_RrMotorAvailTq_Nm]
  [VINP_FrMotorAvailTq_Nm] -> TorqueModule/53(VINP_FrMotorAvailTq_Nm)
  [VINP_RrMotorAvailTq_Nm] -> TorqueModule/54(VINP_RrMotorAvailTq_Nm)
  [task_time_s] -> TorqueModule/55(task_time_s)
  TorqueModule/45(VTQD_LoSpdBrkCtrl_flg) -> VTQD_LoSpdBrkCtrl_flg/1
  TorqueModule/46(VTQD_BOSEnable_flg) -> VTQD_BOSEnable_flg/1
  TorqueModule/52(VTQD_APSStaSys_enum) -> VTQD_APSStaSys_enum/1
  TorqueModule/53(VTQD_APSReq_enum) -> VTQD_APSReq_enum/1
  TorqueModule/54(VTQD_APSDecReqA_flg) -> VTQD_APSDecReqA_flg/1
  TorqueModule/55(VTQD_APSDecReq_mps2) -> VTQD_APSDecReq_mps2/1
  VINP_HSAActive_flg/1 -> [VINP_HSAActive_flg]
  VTQR_NoABSREDUWhlTqReq_Nm/1 -> [VTQR_NoABSREDUWhlTqReq_Nm]
  VTQR_NoABSFEDUWhlTqReq_Nm/1 -> [VTQR_NoABSFEDUWhlTqReq_Nm]
  VINP_AVHActive_flg/1 -> [VINP_AVHActive_flg]
  VINP_DrDoorSW_flg/1 -> [VINP_DrDoorSW_flg]
  VINP_MCUWarnF_enum/1 -> [VINP_MCUWarnF_enum]
  VINP_MCUWarnR_enum/1 -> [VINP_MCUWarnR_enum]
  VVMC_APSSpeedCMD_kph/1 -> [VVMC_APSSpeedCMD_kph]
  VVMC_APSShiftPosnReq_enum/1 -> [VVMC_APSShiftPosnReq_enum]
  VINP_DriverSeatBeltCmd_flg/1 -> [VINP_DriverSeatBeltCmd_flg]
  VINP_ChrgPlugSta_enum/1 -> [VINP_ChrgPlugSta_enum]
  VINP_SeatSW_flg/1 -> [VINP_SeatSW_flg]
  [VINP_MCUWarnF_enum] -> Signal_convert/18(VINP_MCUWarnF_enum)
  [task_time_s] -> Signal_convert/20(task_time_s)
  [VINP_FrEDURealTMTq_Nm] -> Signal_convert/21(VINP_FrEDURealTMTq_Nm)
  [VINP_RrEDURealTMTq_Nm] -> Signal_convert/22(VINP_RrEDURealTMTq_Nm)
  [VINP_MCUWarnR_enum] -> Signal_convert/19(VINP_MCUWarnR_enum)
  [VINP_HSAActive_flg] -> TorqueModule/56(VINP_HSAActive_flg)
  [VTQR_NoABSFEDUWhlTqReq_Nm] -> TorqueModule/57(VTQR_NoABSFEDUWhlTqReq_Nm)
  [VTQR_NoABSREDUWhlTqReq_Nm] -> TorqueModule/58(VTQR_NoABSREDUWhlTqReq_Nm)
  [VINP_AVHActive_flg] -> TorqueModule/59(VINP_AVHActive_flg)
  [VINP_EPBErrSta_enum] -> TorqueModule/60(VINP_EPBErrSta_enum)
  [VINP_MCUWarnF_enum] -> TorqueModule/62(VINP_MCUWarnF_enum)
  [VINP_MCUWarnR_enum] -> TorqueModule/63(VINP_MCUWarnR_enum)
  Signal_convert/17(VTQD_EstVehWeightResult_kg) -> [VTQD_EstVehWeightResult_kg], VTQD_EstVehWeightResult_kg/1
  [VTQD_EPBCarWashMode_flg] -> ShiftModule/8(VTQD_EPBCarWashMode_flg)
  [VINP_DrDoorSW_flg] -> ShiftModule/9(VINP_DrDoorSW_flg)
  [VVMC_APSShiftPosnReq_enum] -> ShiftModule/10(VVMC_APSShiftPosnReq_enum)
  [VVMC_APSActive_flg] -> ShiftModule/11(VVMC_APSActive_flg)
  [VINP_DriverSeatBeltCmd_flg] -> ShiftModule/12(VINP_DriverSeatBeltCmd_flg)
  [VINP_SeatSW_flg] -> ShiftModule/13(VINP_SeatSW_flg)
  [VINP_ChrgPlugSta_enum] -> ShiftModule/14(VINP_ChrgPlugSta_enum)
  [VINP_EPBSta_enum] -> ShiftModule/15(VINP_SCPSystemMode_enum)
  VINP_IVICreepSWReq_flg/1 -> [VINP_IVICreepSWReq_flg]
  TorqueModule/47(VTQD_ExtShftAllow_flg) -> VTQD_ExtShftAllow_flg/1
  TorqueModule/19(VTQD_FrEDUActTqValid_flg) -> Terminator/1
  TorqueModule/20(VTQD_FrEDURolRgnTqValid_flg) -> Terminator1/1
  [VINP_IVICreepSWReq_flg] -> Signal_convert/23(VINP_IVICreepSWReq_flg)
  VPMM_SysPowerMode_enum/1 -> [VPMM_SysPowerMode_enum]
  [VPMM_SysPowerMode_enum] -> Signal_convert/24(VPMM_SysPowerMode_enum)
  TorqueModule/48(VTQD_OPDOn2Off_flg) -> [VTQD_OPDOn2Off_flg]
  [VTQD_OPDOn2Off_flg] -> Signal_convert/25(VTQD_OPDOn2Off_flg)
  [VINP_RegenMode_enum] -> Signal_convert/26(VINP_RegenMode_enum)
  [VTQD_AfterAvailableTqDemFr_Nm] -> ShiftModule/16(VTQD_AfterAvailableTqDemFr_Nm)
  [VTQD_AfterAvailableTqDemRr_Nm] -> ShiftModule/17(VTQD_AfterAvailableTqDemRr_Nm)
  [VTQR_NoABSREDUWhlTqReq_Nm] -> ShiftModule/19(VTQR_NoABSREDUWhlTqReq_Nm)
  [VTQR_NoABSFEDUWhlTqReq_Nm] -> ShiftModule/18(VTQR_NoABSFEDUWhlTqReq_Nm)
  TorqueModule/49(VTQD_PreLoadHold_flg) -> VTQD_PreLoadHold_flg/1
  TorqueModule/50(VTQD_PreLoadPreEn_flg) -> VTQD_PreLoadPreEn_flg/1
  [VINP_DOASta_flg] -> ShiftModule/20(VINP_DOASta_flg)
  VINP_ACCRequiredAccel_mps2/1 -> [VINP_ACCRequiredAccel_mps2]
  [VINP_FrntAxlTrqReqBrk_Nm] -> Signal_convert/27(VINP_FrntAxlTrqReqBrk_Nm)
  [VINP_RearAxlTrqReqBrk_Nm] -> Signal_convert/28(VINP_RearAxlTrqReqBrk_Nm)
  [VINP_FrRBCActive_flg] -> Signal_convert/29(VINP_FrRBCActive_flg)
  [VINP_RrRBCActive_flg] -> Signal_convert/30(VINP_RrRBCActive_flg)
  [VVMC_ADASActive_flg] -> Signal_convert/31(VVMC_ADASActive_flg)
  [VINP_ACCRequiredAccel_mps2] -> Signal_convert/32(VINP_ACCRequiredAccel_mps2)
  TorqueModule/51(VTQD_CreepPrLoadEnable_flg) -> VTQD_CreepPrLoadEnable_flg/1
  Signal_convert/18(VTQD_RDCActive_enum) -> [VTQD_RDCActive_enum], VTQD_RDCActive_enum/1
  VINP_ACCVehHoldReq_flg/1 -> [VINP_ACCVehHoldReq_flg]
  [VINP_ACCVehHoldReq_flg] -> TorqueModule/64(VINP_ACCVehHoldReq_flg)
  VVMC_ACCPedalOvrd_flg/1 -> [VVMC_ACCPedalOvrd_flg]
  [VVMC_ACCPedalOvrd_flg] -> Signal_convert/33(VVMC_ACCPedalOvrd_flg)
  Signal_convert/19(VTQD_EquivAccPedalSWSta_flg) -> VTQD_EquivAccPedalSWSta_flg/1
  ShiftModule/6(VTQD_DriveProtRemove_flg) -> [VTQD_DriveProtRemove_flg]
  [VTQD_DriveProtRemove_flg] -> TorqueModule/65(VTQD_DriveProtRemove_flg)
  [VTQD_AfterAvailableTqDemFr_Nm] -> Signal_convert/34(VTQD_AfterAvailableTqDemFr_Nm)
  [VTQD_AfterAvailableTqDemRr_Nm] -> Signal_convert/35(VTQD_AfterAvailableTqDemRr_Nm)
  ShiftModule/7(VTQD_DriveProtEn_flg) -> VTQD_DriveProtEn_flg/1
  [VINP_ACCRequiredAccel_mps2] -> TorqueModule/66(VINP_ACCRequiredAccel_mps2)
  [VVMC_ADASWhlTqReq_Nm] -> Signal_convert/36(VVMC_ADASWhlTqReq_Nm)
  [VTQR_NoABSREDUWhlTqReq_Nm] -> Signal_convert/37(VTQR_NoABSREDUWhlTqReq_Nm)
  [VTQR_NoABSFEDUWhlTqReq_Nm] -> Signal_convert/38(VTQR_NoABSFEDUWhlTqReq_Nm)
  Signal_convert/20(VTQD_EPBCarWashMode_flg) -> [VTQD_EPBCarWashMode_flg]
  VINP_SCPSystemMode_enum/1 -> [VINP_SCPSystemMode_enum]
  [VTQD_EstVehWeightResult_kg] -> TorqueModule/32(VTQD_EstVehWeightResult_kg)
  [VVMC_LongAcc_Gps] -> TorqueModule/33(VVMC_LongAcc_Gps)
  TorqueModule/56(VTQD_ActParkRequest_flg) -> VTQD_ActParkRequest_flg/1
  VINP_PsngrSeatBeltCmd_flg/1 -> [VINP_PsngrSeatBeltCmd_flg]
  VINP_RDriverSeatBeltCmd_flg/1 -> [VINP_RDriverSeatBeltCmd_flg]
  VINP_RCenterSeatBeltCmd_flg/1 -> [VINP_RCenterSeatBeltCmd_flg]
  VINP_RPsngrSeatBeltCmd_flg/1 -> [VINP_RPsngrSeatBeltCmd_flg]
  VINP_RollModeSWCmd_enum/1 -> [VINP_RollModeSWCmd_enum]
  VVMC_LongAcc_Gps/1 -> [VVMC_LongAcc_Gps]
  VVMC_ActMaxSlideRate_pct/1 -> [VVMC_ActMaxSlideRate_pct]
  VINP_SASAngle_Deg/1 -> [VINP_SASAngle_Deg]
  [VVMC_LongAcc_Gps] -> Signal_convert/39(VVMC_LongAcc_Gps)
  [VINP_DOASta_flg] -> Signal_convert/48(VINP_DOASta_flg)
  [VINP_EPBCarWashMode_flg] -> Signal_convert/47(VINP_EPBCarWashMode_flg)
  [VINP_SCPSystemMode_enum] -> Signal_convert/46(VINP_SCPSystemMode_enum)
  [VINP_RollModeSWCmd_enum] -> Signal_convert/45(VINP_RollModeSWCmd_enum)
  [VINP_RPsngrSeatBeltCmd_flg] -> Signal_convert/44(VINP_RPsngrSeatBeltCmd_flg)
  [VINP_RCenterSeatBeltCmd_flg] -> Signal_convert/43(VINP_RCenterSeatBeltCmd_flg)
  [VINP_RDriverSeatBeltCmd_flg] -> Signal_convert/42(VINP_RDriverSeatBeltCmd_flg)
  [VINP_PsngrSeatBeltCmd_flg] -> Signal_convert/41(VINP_PsngrSeatBeltCmd_flg)
  [VINP_DriverSeatBeltCmd_flg] -> Signal_convert/40(VINP_DriverSeatBeltCmd_flg)
  [VVMC_APSSpeedCMD_kph] -> TorqueModule/61(VVMC_APSSpeedCMD_kph)
  [VVMC_ActMaxSlideRate_pct] -> TorqueModule/52(VVMC_ActMaxSlideRate_pct)
  VVMC_EstSlope_Deg/1 -> [VVMC_EstSlope_Deg]
  [VVMC_EstSlope_Deg] -> Signal_convert/49(VVMC_EstSlope_Deg)
  [VVMC_EstSlope_Deg] -> TorqueModule/67(VVMC_EstSlope_Deg)
  TorqueModule/57(VTQD_RegenTqLimitEn_flg) -> VTQD_RegenTqLimitEn_flg/1
  TorqueModule/58(VTQD_PedAccTqEn_flg) -> VTQD_PedAccTqEn_flg/1
  [VINP_IVIPwrLockSW_enum] -> Signal_convert/50(VINP_IVIPwrLockSW_enum)
  VVMC_RWDRDCActive_enum/1 -> [VVMC_RWDRDCActive_enum]
  VINP_RRDoorSW_flg/1 -> [VINP_RRDoorSW_flg]
  VINP_RLDoorSW_flg/1 -> [VINP_RLDoorSW_flg]
  VINP_HoodSW_flg/1 -> [VINP_HoodSW_flg]
  VINP_TailgateSW_flg/1 -> [VINP_TailgateSW_flg]
  VINP_PsDoorSW_flg/1 -> [VINP_PsDoorSW_flg]
  VINP_IVIPwrLockSW_enum/1 -> [VINP_IVIPwrLockSW_enum]
  Signal_convert/22(VTQD_IVIPwrLockSta_enum) -> VTQD_IVIPwrLockSta_enum/1
  Signal_convert/21(VTQD_IVIPwrLock_flg) -> [VTQD_IVIPwrLock_flg]
  [VTQD_IVIPwrLock_flg] -> ShiftModule/21(VTQD_IVIPwrLock_flg)
  TorqueModule/59(VTQD_ExtDoorAllow_flg) -> VTQD_ExtDoorAllow_flg/1
  VINP_DrSCPSysErrLmp_enum/1 -> [VINP_DrSCPSysErrLmp_enum]
  [VINP_DrDoorSW_flg] -> TorqueModule/68(VINP_DrDoorSW_flg)
  [VINP_PsDoorSW_flg] -> TorqueModule/69(VINP_PsDoorSW_flg)
  [VINP_RRDoorSW_flg] -> TorqueModule/70(VINP_RRDoorSW_flg)
  [VINP_RLDoorSW_flg] -> TorqueModule/71(VINP_RLDoorSW_flg)
  [VINP_HoodSW_flg] -> TorqueModule/72(VINP_HoodSW_flg)
  [VINP_TailgateSW_flg] -> TorqueModule/73(VINP_TailgateSW_flg)
  [VINP_DrSCPSysErrLmp_enum] -> TorqueModule/74(VINP_DrSCPSysErrLmp_enum)
  [VPMM_PowerSta_enum] -> CrashDetect/1(VPMM_PowerSta_enum)
  [VINP_CrashSignalGPIO_flg] -> CrashDetect/2(VINP_CrashSignalGPIO_flg)
  [VINP_CrashOutputSts_enum] -> CrashDetect/3(VINP_CrashOutputSts_enum)
  [task_time_s] -> CrashDetect/4(task_time_s)
  [VINP_EPBSta_enum] -> TorqueModule/75(VINP_EPBSta_enum)
  [VVMC_APSReq_enum] -> TorqueModule/76(VVMC_APSReq_enum)
  VVMC_APSReq_enum/1 -> [VVMC_APSReq_enum]
  [VVMC_RWDRDCActive_enum] -> Signal_convert/51(VVMC_RWDRDCActive_enum)
  [VINP_ADASACCSta_enum] -> TorqueModule/77(VINP_ADASACCSta_enum)
  VINP_ADASACCSta_enum/1 -> [VINP_ADASACCSta_enum]
  TorqueModule/60(VTQD_OPDHoldLamp_flg) -> VTQD_OPDHoldLamp_flg/1
  [VVMC_ActLRSlideRate_pct] -> TorqueModule/78(VVMC_ActLRSlideRate_pct)
  [VVMC_ActRRSlideRate_pct] -> TorqueModule/79(VVMC_ActRRSlideRate_pct)
  [VVMC_ActStESCYaw_degps] -> TorqueModule/80(VVMC_ActStESCYaw_degps)
  VVMC_ActLRSlideRate_pct/1 -> [VVMC_ActLRSlideRate_pct]
  VVMC_ActRRSlideRate_pct/1 -> [VVMC_ActRRSlideRate_pct]
  VVMC_ActStESCYaw_degps/1 -> [VVMC_ActStESCYaw_degps]
  [VINP_SASAngle_Deg] -> TorqueModule/81(VINP_SASAngle_Deg)
  [VINP_YawRate_degps] -> TorqueModule/82(VINP_YawRate_degps)
  VINP_HVBattSOC_pct/1 -> [VINP_HVBattSOC_pct]
  [VINP_HVBattSOC_pct] -> TorqueModule/83(VINP_HVBattSOC_pct)
  TorqueModule/61(VTQD_OPDHoldAllowPark_flg) -> [VTQD_OPDHoldAllowPark_flg]
  [VTQD_OPDHoldAllowPark_flg] -> ShiftModule/22(VTQD_OPDHoldAllowPark_flg)
  Signal_convert/23(VTQD_RegenMode_enum) -> VTQD_RegenMode_enum/1, [VTQD_RegenMode_enum]
  [VVMC_CAASActive_flg] -> TorqueModule/84(VVMC_CAASActive_flg)
  VVMC_CAASActive_flg/1 -> [VVMC_CAASActive_flg]
  TorqueModule/62(VTQD_VehActSpd_kph) -> VTQD_VehActSpd_kph/1
  VVMC_CalibratedGyroY_Dps/1 -> Switch/1
  VINP_YawRate_degps/1 -> Switch/3
  Switch/1 -> [VINP_YawRate_degps]  "VINP_YawRate_degps"
  Constant21/1 -> Switch/2
  TorqueModule/63(VTQD_CreepBaseTqD_Nm) -> VTQD_CreepBaseTqD_Nm/1
  VINP_ABSActive_flg/1 -> [VINP_ABSActive_flg]
  VINP_ESCActive_flg/1 -> [VINP_ESCActive_flg]
  [VINP_ABSActive_flg] -> TorqueModule/85(VINP_ABSActive_flg)
  [VINP_ESCActive_flg] -> TorqueModule/86(VINP_ESCActive_flg)

== system tqd/TQD/TorqueDemand/CrashDetect ==
  VPMM_PowerSta_enum : Inport
  VINP_CrashSignalGPIO_flg : Inport  Port=2
  VINP_CrashOutputSts_enum : Inport  Port=3
  task_time_s : Inport  Port=4
  Add1 : Sum
  Add2 : Sum
  Add3 : Sum
  Constant1 : Constant  Value=ENUM_POWERSTA_ON
  Constant{3,8,10,19,23,36} (6 alike) : Constant  Value=KTQD_CrashPWMCnt_cnt
  Constant{6,11,20,26,31,34} (6 alike) : Constant  Value=ZERO_INT
  Constant12 : Constant  Value=KTQD_50MS_cnt
  Constant13 : Constant  Value=KTQD_PwrStaTimerforCrash_s
  Constant14 : Constant  Value=ENUM_CRASHSTATE_NOCRASH
  Constant15 : Constant  Value=KTQD_DiagHCrashTimer_s
  Constant16 : Constant  Value=ENUM_CRASHSTATE_NOCRASH
  Constant17 : Constant  Value=ENUM_CRASHSTATE_NOCRASH
  Constant18 : Constant  Value=KTQD_PwrStaTimerforCrash_s
  Constant2 : Constant  Value=ENUM_POWERSTA_READY
  Constant21 : Constant  Value=KTQD_50MS_cnt
  Constant22 : Constant  Value=ZERO_FLOAT
  Constant24 : Constant  Value=KTQD_NoDiagHCrashTimer_s
  Constant25 : Constant  Value=KTQD_DiagHCrashTimer_s
  Constant27 : Constant  Value=KTQD_190MS_cnt
  Constant28 : Constant  Value=KTQD_30MS_cnt
  Constant29 : Constant  Value=KTQD_50MS_cnt
  Constant30 : Constant  Value=KTQD_210MS_cnt
  Constant32 : Constant  Value=KTQD_NoDiagHCrashTimer_s
  Constant35 : Constant  Value=KTQD_210MS_cnt
  Constant4 : Constant  Value=ONE_INT
  Constant5 : Constant  Value=ENUM_POWERSTA_OFF
  Constant7 : Constant  Value=KTQD_210MS_cnt
  Constant9 : Constant  Value=FALSE
  Data Type Conversion1 : DataTypeConversion
  Data Type Conversion2 : DataTypeConversion
  Equal : RelationalOperator  Operator=~=  OutDataTypeStr=boolean  RndMeth=Simplest
  Equal{1..2,6,10} (4 alike) : RelationalOperator  Operator===  OutDataTypeStr=boolean  RndMeth=Simplest
  Equal{3,7,9,11,13} (5 alike) : RelationalOperator  OutDataTypeStr=boolean  RndMeth=Simplest
  Equal12 : RelationalOperator  Operator=<  OutDataTypeStr=boolean  RndMeth=Simplest
  Equal4 : RelationalOperator  Operator=~=  OutDataTypeStr=boolean  RndMeth=Simplest
  Equal5 : RelationalOperator  Operator=<  OutDataTypeStr=boolean  RndMeth=Simplest
  Equal8 : RelationalOperator  Operator=~=  OutDataTypeStr=boolean  RndMeth=Simplest
  Logical Operator{,9..10,13,16,21} (6 alike) : Logic  Operator=OR  AllPortsSameDT=off  OutDataTypeStr=boolean
  Logical Operator{1,3,7..8,18,20} (6 alike) : Logic  Operator=NOT  AllPortsSameDT=off  OutDataTypeStr=boolean
  Logical Operator{4..5,11..12,14..15,17,19} (8 alike) : Logic  AllPortsSameDT=off  OutDataTypeStr=boolean
  Logical Operator2 : Logic  Inputs=3  AllPortsSameDT=off  OutDataTypeStr=boolean
  Logical Operator6 : Logic  Inputs=3  AllPortsSameDT=off  OutDataTypeStr=boolean
  Relational Operator{,5..7,9} (5 alike) : RelationalOperator  Operator=>  OutDataTypeStr=boolean  RndMeth=Simplest
  Relational Operator1 : RelationalOperator  OutDataTypeStr=boolean  RndMeth=Simplest
  Relational Operator10 : RelationalOperator  Operator=<  OutDataTypeStr=boolean  RndMeth=Simplest
  Relational Operator2 : RelationalOperator  Operator=<=  OutDataTypeStr=boolean  RndMeth=Simplest
  Relational Operator3 : RelationalOperator  OutDataTypeStr=boolean  RndMeth=Simplest
  Relational Operator4 : RelationalOperator  Operator=<=  OutDataTypeStr=boolean  RndMeth=Simplest
  Relational Operator8 : RelationalOperator  Operator=<  OutDataTypeStr=boolean  RndMeth=Simplest
  SR_Latch : hcu_lib/Basic_Blocks/SR_Latch
  Switch1 : Switch  Criteria=u2 ~= 0
  Switch{2..9} (8 alike) : Switch  Criteria=u2 > Threshold
  Timer2 : hcu_lib/Basic_Blocks/Timer
  Timer3 : hcu_lib/Basic_Blocks/Timer
  Timer4 : hcu_lib/Basic_Blocks/Timer
  Unit Delay{1..3,5} (4 alike) : UnitDelay  SampleTime=-1  HasFrameUpgradeWarning=on
  VTQD_CrashDetd_flg : Outport
  VTQD_DiagHCrash_flg : Outport  Port=2
  wires:
  [VPMM_PowerSta_enum] -> Equal2/1
  Logical Operator/1 -> Logical Operator3/1, Timer2/1
  [VPMM_PowerSta_enum] -> Equal1/1
  Constant13/1 -> Equal7/2
  Timer2/1 -> Equal7/1
  Constant18/1 -> Timer2/4
  Logical Operator3/1 -> Timer2/2
  Constant1/1 -> Equal1/2
  Constant2/1 -> Equal2/2
  Equal7/1 -> [VTQD_PwrStaTimerReady_flg]  "VTQD_PwrStaTimerReady_flg"
  [task_time_s] -> Timer2/3
  VPMM_PowerSta_enum/1 -> [VPMM_PowerSta_enum]
  VINP_CrashSignalGPIO_flg/1 -> [VINP_CrashSignalGPIO_flg]
  Equal1/1 -> Logical Operator/1
  Equal2/1 -> Logical Operator/2
  VINP_CrashOutputSts_enum/1 -> [VINP_CrashOutputSts_enum]
  Constant15/1 -> Equal11/2
  Timer3/1 -> Equal11/1
  Logical Operator7/1 -> Timer3/2
  Constant25/1 -> Timer3/4
  [task_time_s] -> Timer3/3
  [VTQD_CrashOutputSts_flg] -> Logical Operator7/1, Timer3/1
  task_time_s/1 -> [task_time_s]
  Data Type Conversion1/1 -> Add3/2
  Constant8/1 -> Relational Operator8/2
  Relational Operator8/1 -> Data Type Conversion1/1
  [VTQD_CrashCountEN_flg] -> Switch6/2
  [VTQD_PwrStaTimerReady_flg] -> Switch7/2
  Constant29/1 -> Relational Operator2/2
  Unit Delay3/1 -> Equal/1
  Constant26/1 -> Switch7/3
  Switch6/1 -> Switch3/1
  Logical Operator10/1 -> [VTQD_CrashCountEN_flg]
  Constant22/1 -> Relational Operator/2
  Add2/1 -> Switch2/3
  [VTQD_CrashChange_flg] -> Switch3/2
  Logical Operator6/1 -> Logical Operator10/2
  Constant28/1 -> Relational Operator1/2
  Logical Operator2/1 -> Logical Operator10/1
  Switch3/1 -> Switch7/1
  Equal/1 -> [VTQD_CrashChange_flg]
  Add3/1 -> Switch6/1
  Relational Operator3/1 -> Logical Operator6/2
  Constant6/1 -> Switch6/3
  Constant4/1 -> Add2/2
  Relational Operator2/1 -> Logical Operator2/3
  Logical Operator1/1 -> Logical Operator2/1
  [VTQD_fCrash_cnt] -> Relational Operator8/1, Add3/1
  Switch2/1 -> Unit Delay1/1
  Unit Delay5/1 -> [VTQD_fCrash_cnt], Equal3/1  "VTQD_fCrash_cnt"
  Relational Operator/1 -> Equal/2, Unit Delay3/1
  [VTQD_CrashChange_flg] -> Switch2/2
  [VINP_CrashSignalGPIO_flg] -> Logical Operator1/1
  [VTQD_CrashCount_enum] -> Relational Operator2/1, Relational Operator1/1
  Relational Operator1/1 -> Logical Operator2/2
  Constant31/1 -> Switch2/1
  [VINP_CrashSignalGPIO_flg] -> Relational Operator/1
  Constant10/1 -> Equal3/2
  [VTQD_PwrStaTimerReady_flg] -> Logical Operator12/2
  Logical Operator12/1 -> Logical Operator13/2, [VTQD_CrashOutputSts_flg]
  Equal4/1 -> Logical Operator12/1
  Constant14/1 -> Equal4/2
  [VINP_CrashOutputSts_enum] -> Equal4/1
  Switch7/1 -> Unit Delay5/1
  Unit Delay1/1 -> [VTQD_CrashCount_enum]
  [VTQD_CrashCount_enum] -> Add2/1
  Logical Operator4/1 -> Logical Operator9/2
  [VTQD_CrashCount_enum] -> Relational Operator6/1
  Relational Operator6/1 -> Logical Operator4/2
  [VINP_CrashSignalGPIO_flg] -> Logical Operator8/1
  Logical Operator5/1 -> Logical Operator9/1
  Constant7/1 -> Relational Operator6/2
  Constant11/1 -> Switch4/1
  Logical Operator8/1 -> Logical Operator4/1
  [VTQD_fCrash_cnt] -> Switch4/3
  [VTQD_CrashCount_enum] -> Relational Operator7/1
  Logical Operator9/1 -> Switch4/2
  Relational Operator7/1 -> Logical Operator5/2
  [VINP_CrashSignalGPIO_flg] -> Logical Operator5/1
  Constant12/1 -> Relational Operator7/2
  Switch4/1 -> Switch3/3
  Equal3/1 -> Logical Operator13/1
  Logical Operator13/1 -> VTQD_CrashDetd_flg/1  "VTQD_CrashDetd_flg"
  [VINP_CrashSignalGPIO_flg] -> Logical Operator6/1
  Relational Operator4/1 -> Logical Operator6/3
  Constant30/1 -> Relational Operator4/2
  Constant27/1 -> Relational Operator3/2
  [VTQD_CrashCount_enum] -> Relational Operator4/1, Relational Operator3/1
  Constant3/1 -> Equal5/2
  [VTQD_fCrash_cnt] -> Equal5/1
  Equal5/1 -> Logical Operator11/1
  Equal11/1 -> Logical Operator11/2
  SR_Latch/1 -> VTQD_DiagHCrash_flg/1  "VTQD_DiagHCrash_flg"
  Logical Operator11/1 -> SR_Latch/1
  Constant5/1 -> Equal6/2
  [VPMM_PowerSta_enum] -> Equal6/1
  Equal6/1 -> Switch1/2
  Switch1/1 -> SR_Latch/2
  Constant9/1 -> Switch1/1
  Constant19/1 -> Equal9/2
  Equal9/1 -> Logical Operator14/1
  Logical Operator16/1 -> Logical Operator18/1, Timer4/1
  Logical Operator14/1 -> Logical Operator16/1
  Constant23/1 -> Equal12/2
  Equal12/1 -> Logical Operator17/1
  Logical Operator17/1 -> Logical Operator16/2
  Timer4/1 -> Equal13/1
  Equal13/1 -> Switch1/3
  Constant24/1 -> Equal13/2
  Constant32/1 -> Timer4/4
  [task_time_s] -> Timer4/3
  Logical Operator18/1 -> Timer4/2
  [VINP_CrashOutputSts_enum] -> Equal8/1
  Constant16/1 -> Equal8/2
  Equal8/1 -> Logical Operator14/2
  [VINP_CrashOutputSts_enum] -> Equal10/1
  Equal10/1 -> Logical Operator17/2
  Constant17/1 -> Equal10/2
  [test_crash_cnt] -> Switch8/3
  Constant35/1 -> Relational Operator5/2
  [VTQD_CrashCount_enum] -> Relational Operator5/1
  Constant21/1 -> Relational Operator9/2
  [VTQD_CrashCount_enum] -> Relational Operator9/1
  [VINP_CrashSignalGPIO_flg] -> Logical Operator19/1
  Relational Operator9/1 -> Logical Operator19/2
  Logical Operator15/1 -> Logical Operator21/2
  [VINP_CrashSignalGPIO_flg] -> Logical Operator20/1
  Logical Operator20/1 -> Logical Operator15/1
  Constant20/1 -> Switch8/1
  Logical Operator19/1 -> Logical Operator21/1
  Add1/1 -> Switch9/1
  Relational Operator5/1 -> Logical Operator15/2
  Constant34/1 -> Switch9/3
  Logical Operator21/1 -> Switch8/2
  Switch5/1 -> Unit Delay2/1
  [test_crash_cnt] -> Relational Operator10/1, Add1/1
  Constant36/1 -> Relational Operator10/2
  Relational Operator10/1 -> Data Type Conversion2/1
  Switch8/1 -> Switch5/3
  [VTQD_CrashChange_flg] -> Switch5/2
  Data Type Conversion2/1 -> Add1/2
  Switch9/1 -> Switch5/1
  [VTQD_CrashCountEN_flg] -> Switch9/2
  Unit Delay2/1 -> Equal9/1, Equal12/1, [test_crash_cnt]
